simulink model "simple_pendulam"  (R2021a)
settings: Solver=VariableStepAuto  StartTime=0.0  StopTime=10.0  RelTol=1e-3
InitFcn:
  | g=9.8
  | l=2
  | theta = 40
settings Model: Creator=DELL  LastModifiedBy=DELL

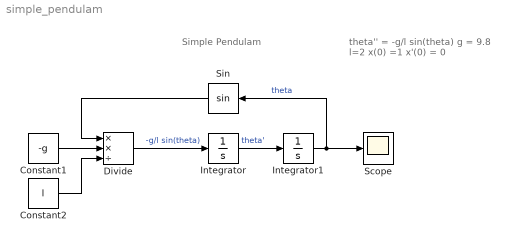
== system simple_pendulam ==
  note: Simple Pendulam
  note: theta'' = -g/l sin(theta)
      | g = 9.8 l=2
      | x(0) =1
      | x'(0) = 0
  Constant1 : Constant  Value=-g
  Constant2 : Constant  Value=l
  Divide : Product  Inputs=**/
  Integrator : Integrator
  Integrator1 : Integrator  InitialCondition=1
  Scope : Scope
  Sin : Trigonometry
  wires:
  Integrator/1 -> Integrator1/1  "theta'"
  Constant2/1 -> Divide/3
  Constant1/1 -> Divide/2
  Divide/1 -> Integrator/1  "-g/l sin(theta)"
  Integrator1/1 -> Sin/1, Scope/1  "theta"
  Sin/1 -> Divide/1
